simulink model "Deadzone"  (R2017b)
settings: Solver=ode3  StartTime=0.0  StopTime=10.0  FixedStep=0.200000  RelTol=1e-3  EnableMultiTasking=on
settings Model: Creator=hbourbou  LastModifiedBy=hbourbou
settings DataIOCC: LimitDataPoints=on  SaveFormat=Structure
settings OptimizationCC: LifeSpan=inf
settings DebuggingCC: SFUnexpectedBacktrackingDiag=warning  SFNoUnconditionalDefaultTransitionDiag=warning  SFExecutionAtInitializationDiag=none
settings HardwareCC: ProdBitPerPointer=32  ProdBitPerSizeT=32  ProdBitPerPtrDiffT=32  ProdLargestAtomicFloat=None  ProdIntDivRoundTo=Undefined  ProdEndianess=Unspecified  ProdWordSize=32  ProdHWDeviceType=32-bit Generic
settings ModelReferenceCC: PropagateSignalLabelsOutOfModel=off
settings CodeAppCC: StateflowObjectComments=on
settings GRTTargetCC: TargetLangStandard=C89/C90 (ANSI)  GeneratePreprocessorConditionals=Disable all
settings ConfigComp: CovMetricSettings=dw  CovHtmlReporting=on  CovSaveCumulativeToWorkspaceVar=on  CovSaveSingleToWorkspaceVar=on  CovExternalEMLEnable=off

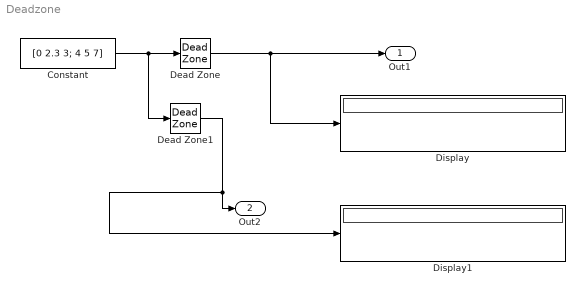
== system Deadzone ==
  Constant : Constant  Value=[0 2.3 3; 4 5 7]
  Dead Zone : DeadZone  LowerValue=2  UpperValue=5  SaturateOnIntegerOverflow=on
  Dead Zone1 : DeadZone  LowerValue=2  UpperValue=5  SaturateOnIntegerOverflow=on
  Display : Display
  Display1 : Display
  Out1 : Outport
  Out2 : Outport  Port=2
  wires:
  Constant/1 -> Dead Zone1/1, Dead Zone/1
  Dead Zone/1 -> Display/1, Out1/1
  Dead Zone1/1 -> Display1/1, Out2/1
